simulink model "filter_test"  (R2015a)
settings: Solver=ode45  StartTime=0.0  StopTime=5  RelTol=1e-3
values from neighbouring files (symbols this model uses):
  anpha_0 = 5    [ANN_params.m]    (also in furuta.m)
  beta0 = 5.8*10^(-4)    (= 0.00058)    [ANN_params.m]    (also in furuta.m)
  beta1 = 1.4142*10^(-3)    (= 0.0014142)    [ANN_params.m]    (also in furuta.m)
  c = 10    [ANN_params.m]
  g = 9.81    [ANN_params.m]    (also in furuta.m)
  J0 = 4.4*10^(-3)    (= 0.0044)    [ANN_params.m]    (also in furuta.m)
  J1 = 5.5026*10^(-4)    (= 0.00055026)    [ANN_params.m]    (also in furuta.m)
  k = 3    [ANN_params.m]
  L0 = 0.157    [ANN_params.m]    (also in furuta.m)
  L1 = 0.133    [ANN_params.m]    (also in furuta.m)
  m1 = 0.078    [ANN_params.m]    (also in furuta.m = 0.0933)
  theta_0 = 0    [ANN_params.m]    (also in furuta.m)
settings Model: Creator=chech  LastModifiedBy=chech
settings SolverCC: ZeroCrossAlgorithm=Adaptive

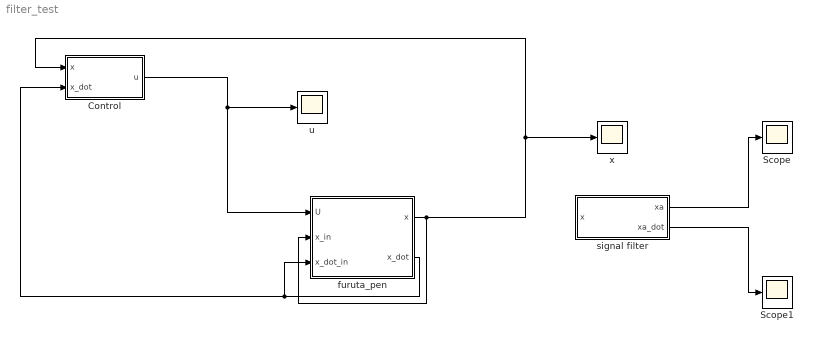
== system filter_test ==
  Control : Subsystem
  Scope : Scope
      settings: YMin=-0.5  YMax=5.25
  Scope1 : Scope
      settings: TimeRange=5  YMin=-20  YMax=27.5
  furuta_pen : Subsystem
  signal filter : Subsystem
  u : Scope
      settings: YMin=-4.5  YMax=3  SaveName=ScopeData3
  x : Scope
      settings: YMin=-4.5  YMax=0.25  SaveName=ScopeData2
  wires:
  furuta_pen/2(x_dot) -> Control/2(x_dot), furuta_pen/3(x_dot_in)
  furuta_pen/1(x) -> furuta_pen/2(x_in), x/1, Control/1(x)
  signal filter/1(xa) -> Scope/1
  signal filter/2(xa_dot) -> Scope1/1
  Control/1(u) -> u/1, furuta_pen/1(U)

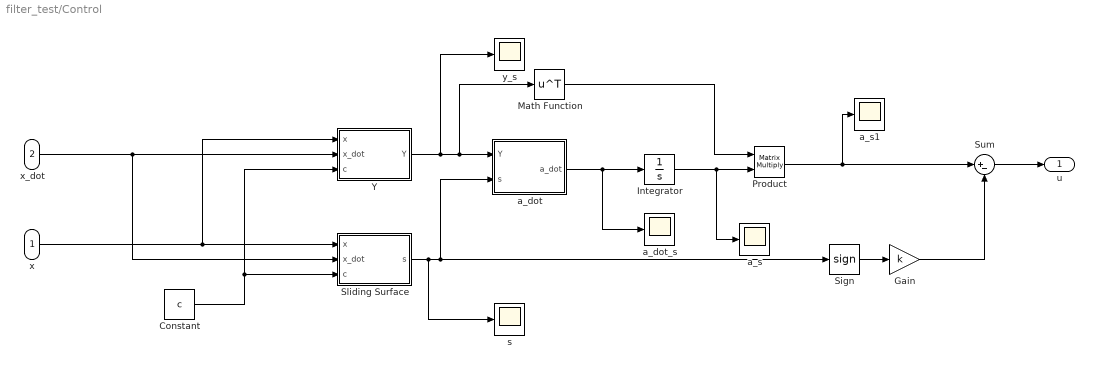
== system filter_test/Control ==
  x : Inport
  x_dot : Inport  Port=2
  Constant : Constant  Value=c
  Gain : Gain  Gain=k
  Integrator : Integrator  InitialCondition=[0.5;0.5;0.5;0.5]
  Math Function : Math  Operator=transpose  SaturateOnIntegerOverflow=on
  Product : Product  Multiplication=Matrix(*)
  Sign : Signum
  Sliding Surface : MATLAB Function  TreatAsAtomicUnit=on
  Sum : Sum  Inputs=|+-
  Y : MATLAB Function  TreatAsAtomicUnit=on
  a_dot : MATLAB Function  TreatAsAtomicUnit=on
  a_dot_s : Scope
      settings: YMin=-0.175  YMax=0.175  SaveName=ScopeData6
  a_s : Scope
      settings: YMin=0.491  YMax=0.504  SaveName=ScopeData7
  a_s1 : Scope
      settings: YMin=0.491  YMax=0.504  SaveName=ScopeData8
  s : Scope
      settings: YMin=-0.175  YMax=0.175  SaveName=ScopeData5
  y_s : Scope
      settings: YMin=-0.175  YMax=0.175  SaveName=ScopeData4
  u : Outport
  wires:
  x_dot/1 -> Sliding Surface/2(x_dot), Y/2(x_dot)
  x/1 -> Y/1(x), Sliding Surface/1(x)
  Constant/1 -> Sliding Surface/3(c), Y/3(c)
  a_dot/1(a_dot) -> a_dot_s/1, Integrator/1
  Y/1(Y) -> y_s/1, Math Function/1, a_dot/1(Y)
  Sliding Surface/1(s) -> s/1, a_dot/2(s), Sign/1
  Math Function/1 -> Product/1
  Integrator/1 -> a_s/1, Product/2
  Product/1 -> a_s1/1, Sum/1
  Sign/1 -> Gain/1
  Gain/1 -> Sum/2
  Sum/1 -> u/1

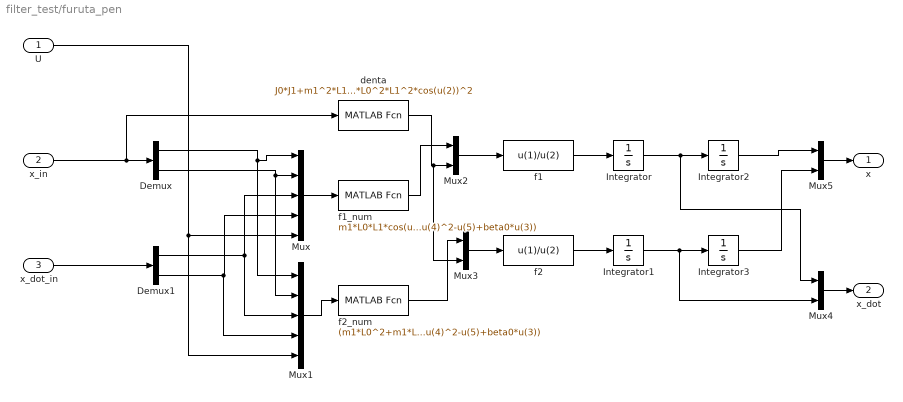
== system filter_test/furuta_pen ==
  U : Inport
  x_in : Inport  Port=2
  x_dot_in : Inport  Port=3
  Demux : Demux  Outputs=2
  Demux1 : Demux  Outputs=2
  Integrator : Integrator
  Integrator1 : Integrator
  Integrator2 : Integrator  InitialCondition=theta_0*pi/180
  Integrator3 : Integrator  InitialCondition=anpha_0/180*pi
  Mux : Mux  Inputs=5
  Mux1 : Mux  Inputs=5
  Mux{2..5} (4 alike) : Mux  Inputs=2
  denta : MATLABFcn  MATLABFcn=J0*J1+m1^2*L1^4*sin(u(2))^2+m1^2*L0^2*L1^2+J0*m1*L1^2+J1*m1*L0^2+J1*m1*L1^2*sin(u(2))^2-m1^2*L0^2*L1^2*cos(u(2))^2  OutputDimensions=1
  f1 : MATLABFcn  MATLABFcn=u(1)/u(2)  OutputDimensions=1
  f1_num : MATLABFcn  MATLABFcn=m1*L0*L1*cos(u(2))*(0.5*m1*L1^2*sin(2*u(2))*u(3)^2+m1*g*L1*sin(u(2))-beta1*u(4))-(m1*L1^2+J1)*(m1*L1^2*sin(2*u(2))*u(3)*u(4)+m1*L0*L1*sin(u(2))*u(4)^2-u(5)+beta0*u(3))  OutputDimensions=1
  f2 : MATLABFcn  MATLABFcn=u(1)/u(2)  OutputDimensions=1
  f2_num : MATLABFcn  MATLABFcn=(m1*L0^2+m1*L1^2*sin(u(2))^2+J0)*(0.5*m1*L1^2*sin(2*u(2))*u(3)^2+m1*g*L1*sin(u(2))-beta1*u(4))-m1*L0*L1*cos(u(2))*(m1*L1^2*sin(2*u(2))*u(3)*u(4)+m1*L0*L1*sin(u(2))*u(4)^2-u(5)+beta0*u(3))  OutputDimensions=1
  x : Outport
  x_dot : Outport  Port=2
  wires:
  x_in/1 -> Demux/1, denta/1
  Mux/1 -> f1_num/1
  Mux1/1 -> f2_num/1
  Mux2/1 -> f1/1
  denta/1 -> Mux3/2, Mux2/2
  f1_num/1 -> Mux2/1
  Mux3/1 -> f2/1
  f2_num/1 -> Mux3/1
  f1/1 -> Integrator/1
  f2/1 -> Integrator1/1
  Integrator/1 -> Mux4/1, Integrator2/1
  Integrator1/1 -> Mux4/2, Integrator3/1
  Mux4/1 -> x_dot/1
  Mux5/1 -> x/1
  Integrator2/1 -> Mux5/1
  Integrator3/1 -> Mux5/2
  U/1 -> Mux1/5, Mux/5
  x_dot_in/1 -> Demux1/1
  Demux/1 -> Mux1/1, Mux/1
  Demux/2 -> Mux1/2, Mux/2
  Demux1/2 -> Mux1/4, Mux/4
  Demux1/1 -> Mux1/3, Mux/3

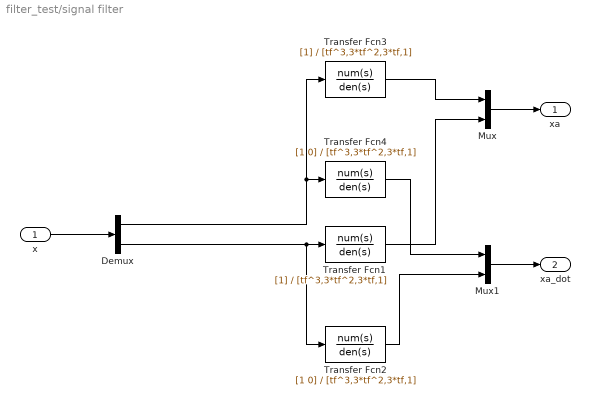
== system filter_test/signal filter ==
  x : Inport
  Demux : Demux  Outputs=2
  Mux : Mux  Inputs=2
  Mux1 : Mux  Inputs=2
  Transfer Fcn1 : TransferFcn  Denominator=[tf^3,3*tf^2,3*tf,1]
  Transfer Fcn2 : TransferFcn  Numerator=[1 0]  Denominator=[tf^3,3*tf^2,3*tf,1]
  Transfer Fcn3 : TransferFcn  Denominator=[tf^3,3*tf^2,3*tf,1]
  Transfer Fcn4 : TransferFcn  Numerator=[1 0]  Denominator=[tf^3,3*tf^2,3*tf,1]
  xa : Outport
  xa_dot : Outport  Port=2
  wires:
  Demux/1 -> Transfer Fcn3/1, Transfer Fcn4/1
  x/1 -> Demux/1
  Transfer Fcn4/1 -> Mux1/1
  Demux/2 -> Transfer Fcn2/1, Transfer Fcn1/1
  Mux1/1 -> xa_dot/1
  Transfer Fcn2/1 -> Mux1/2
  Transfer Fcn3/1 -> Mux/1
  Transfer Fcn1/1 -> Mux/2
  Mux/1 -> xa/1

== matlab function filter_test/Control/Y ==
  data: x input size=2; Y output; x_dot input size=2; c input size=1
function Y = fnc(x,x_dot,c)
%#codegen

Y = [-c*x_dot(2);x_dot(2);x(2);x_dot(1)];

== matlab function filter_test/Control/Sliding Surface ==
  data: x input size=2; s output size=1; x_dot input size=2; c input size=1
function s = fcn(x,x_dot,c)
%#codegen
s = x_dot(2)+c*x(2);

== matlab function filter_test/Control/a_dot ==
  data: Y input size=4; s input size=1; a_dot output
function a_dot = fnc(Y,s)
%#codegen
ro = 100*eye(4);
a_dot = -ro^(-1)*Y*s;
